simulink model "Srm_dtc"  (Simulink 8.5)
settings: Solver=FixedStepDiscrete  StartTime=0.0  StopTime=1  FixedStep=Ts  RelTol=1e-3  AbsTol=1e-5
PreLoadFcn:
  | Ts=1e-5;
  | load srm64_60kw
undefined symbols (not defined in the file or in its folder): find_system, magnitude
libraries: powerlib x15, simulink x1
Description:
  | Copyright 2008-2010 The MathWorks, Inc.
settings Model: Creator=MathWorks  LastModifiedBy=think0404  ExtModeAutoUpdateStatusClock=off
settings DataIOCC: SignalLoggingName=sigsOut
settings OptimizationCC: InitFltsAndDblsToZero=on
settings DebuggingCC: CheckExecutionContextPreStartOutputMsg=on  CheckExecutionContextRuntimeOutputMsg=on  SignalResolutionControl=TryResolveAllWithWarning  MultiTaskDSMMsg=warning  MultiTaskCondExecSysMsg=none  FcnCallInpInsideContextMsg=UseLocalSettings
settings HardwareCC: TargetUnknown=on

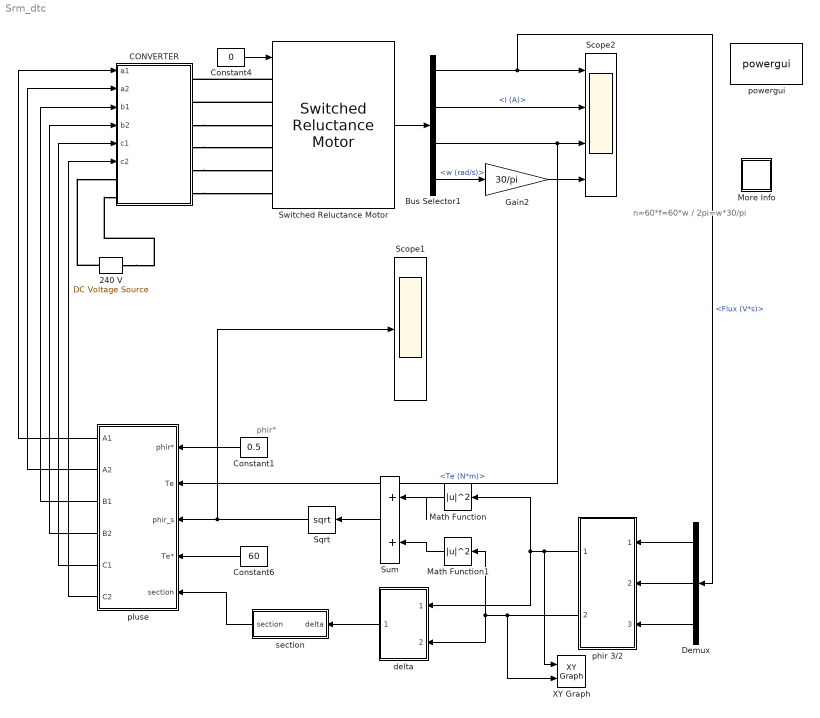
== system Srm_dtc ==
  note: phir*
  note: n=60*f=60*w / 2pi=w*30/pi
  " phir 3/2" : Subsystem
  240 V : powerlib/Electrical Sources/DC Voltage Source  Amplitude=300  Measurements=None
  Bus Selector1 : BusSelector  OutputSignals=Flux (V*s),I (A),Te (N*m),w (rad/s)
  CONVERTER : Subsystem  LoadFcn=find_system(gcs,'FollowLinks', 'on', 'LookUnderMasks', 'all');
  Constant1 : Constant  Value=0.5
  Constant4 : Constant  Value=0
  Constant6 : Constant  Value=60
  Demux : Demux  Outputs=3
  Gain2 : Gain  Gain=30/pi  SaturateOnIntegerOverflow=on  OutDataTypeStr=Inherit: Same as input  ParamDataTypeStr=Inherit: Same as input
  Math Function : Math  Operator=magnitude^2  SaturateOnIntegerOverflow=on
  Math Function1 : Math  Operator=magnitude^2  SaturateOnIntegerOverflow=on
  More Info : Subsystem  Description=asb
      settings: OpenFcn=showdemo(bdroot(gcb))
      mask Display: disp('?')
  Scope1 : Scope
      settings: TimeRange=0.1  YMin=-0.05  YMax=0.55  SaveName=VI1  Decimation=10
  Scope2 : Scope  NumInputPorts=4
      settings: TimeRange=0.1  YMin=-0.05~-100~-20~-10  YMax=0.55~800~70~90  SaveName=VI  Decimation=10
  Sqrt : Sqrt  SaturateOnIntegerOverflow=on
  Sum : Sum  Inputs=|++
  Switched Reluctance Motor : powerlib/Machines/Switched Reluctance Motor  MachineType=6/4  StatorResistance=0.05  Inertia=0.05  Friction=0.02  InitialSpeed=[0,0]  TsPowergui=0  TsBlock=-1  MachineModel=Generic model  Lq=0.67e-3  Ld=23.6e-3  Lsat=0.15e-3  MaximumCurrent=450  MaximumFluxLinkage=0.486  Source=MAT-file  MagnetisationCharacteristic='srm64_60kw.mat'  RotorAngleVector=[0 10 20 30 40 45]  StatorCurrentVector=0:25:450  PlotCurves=off
  XY Graph : simulink/Sinks/XY Graph  xmin=-1  xmax=1  ymin=-1  ymax=1  st=-1
  "delta " : Subsystem
  pluse : Subsystem
  powergui : powerlib/powergui  Priority=2  SimulationMode=Discrete  SolverType=Tustin/Backward Euler (TBE)  SampleTime=Ts  frequency=60  SPID=off  DisableSnubberDevices=off  DisableRonSwitches=off  DisableVfSwitches=off  SwTol=0  DisplayEquations=off  Interpol=off  methode=off  Ts=0  FunctionMessages=off  echomessages=off  HookPort=off  EnableUseOfTLC=off  x0status=blocks  frequencyindice=0  Pbase=100e6  ErrMax=1e-4  Iterations=50  UnitsV=kV  UnitsW=MW  buscounter=0  RestoreLinks=warning  ResistiveCurrentMeasurement=off  Frange=[0:2:500]  Ylog=off  Xlog=on  ShowGrid=off  save=off  variable=ZData  structure=0  ZoomFFT=on  StartTime=0.0  cycles=1  DisplayStyle=1  fundamental=60  FreqAxis=off  MaxFrequency=1000  frequencyindicesteady=1  RmsSteady=1  display=off
  "section " : Subsystem
  wires:
  Constant4/1 -> Switched Reluctance Motor/1
  Switched Reluctance Motor/1 -> Bus Selector1/1
  Bus Selector1/1 -> Scope2/1, Demux/1  "<Flux (V*s)>"
  Bus Selector1/2 -> Scope2/2  "<I (A)>"
  Bus Selector1/3 -> Scope2/3, pluse/2(Te)  "<Te (N*m)>"
  Gain2/1 -> Scope2/4
  Bus Selector1/4 -> Gain2/1  "<w (rad/s)>"
  Demux/1 -> " phir 3/2"/1(phir_a)
  Demux/2 -> " phir 3/2"/2(phir_b)
  Demux/3 -> " phir 3/2"/3(phir_c)
  " phir 3/2"/1(phir_alpha) -> Math Function/1, "delta "/1(phir_alpha), XY Graph/1
  " phir 3/2"/2(phir_beta) -> Math Function1/1, "delta "/2(phir_beta), XY Graph/2
  Math Function/1 -> Sum/1
  Math Function1/1 -> Sum/2
  Sum/1 -> Sqrt/1
  "delta "/1(delta) -> "section "/1(delta)
  Sqrt/1 -> pluse/3(phir_s), Scope1/1
  Constant1/1 -> pluse/1(phir*)
  Constant6/1 -> pluse/4(Te*)
  "section "/1(section) -> pluse/5(section)
  pluse/1(A1) -> CONVERTER/1(a1)
  pluse/2(A2) -> CONVERTER/2(a2)
  pluse/3(B1) -> CONVERTER/3(b1)
  pluse/4(B2) -> CONVERTER/4(b2)
  pluse/5(C1) -> CONVERTER/5(c1)
  pluse/6(C2) -> CONVERTER/6(c2)
  connections:
  Switched Reluctance Motor/LConn1 -- CONVERTER/RConn1
  Switched Reluctance Motor/LConn2 -- CONVERTER/RConn2
  CONVERTER/RConn3 -- Switched Reluctance Motor/LConn3
  CONVERTER/RConn4 -- Switched Reluctance Motor/LConn4
  CONVERTER/RConn5 -- Switched Reluctance Motor/LConn5
  CONVERTER/RConn6 -- Switched Reluctance Motor/LConn6
  240 V/RConn1 -- CONVERTER/LConn1
  240 V/LConn1 -- CONVERTER/LConn2

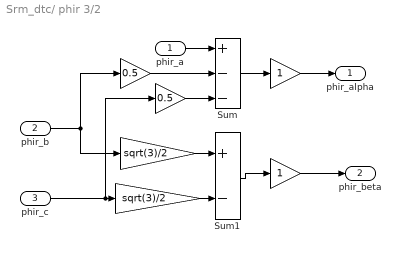
== system Srm_dtc/ phir 3/2 ==
  phir_a : Inport
  phir_b : Inport  Port=2
  phir_c : Inport  Port=3
  " " : Gain  Gain=0.5
  "   " : Gain  Gain=0.5
  "    " : Gain  Gain=sqrt(3)/2
  "     " : Gain  Gain=sqrt(3)/2
  "          " : Gain
  "              " : Gain
  Sum : Sum  Inputs=+--
  Sum1 : Sum  Inputs=+-
  phir_alpha : Outport
  phir_beta : Outport  Port=2
  wires:
  phir_a/1 -> Sum/1
  " "/1 -> Sum/2
  "   "/1 -> Sum/3
  "     "/1 -> Sum1/1
  "    "/1 -> Sum1/2
  phir_b/1 -> " "/1, "     "/1
  phir_c/1 -> "   "/1, "    "/1
  Sum/1 -> "          "/1
  Sum1/1 -> "              "/1
  "          "/1 -> phir_alpha/1
  "              "/1 -> phir_beta/1

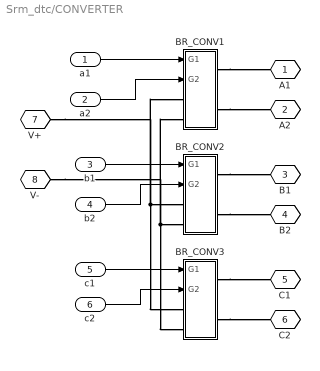
== system Srm_dtc/CONVERTER ==
  a1 : Inport
  a2 : Inport  Port=2
  b1 : Inport  Port=3
  b2 : Inport  Port=4
  c1 : Inport  Port=5
  c2 : Inport  Port=6
  BR_CONV1 : Subsystem
  BR_CONV2 : Subsystem
  BR_CONV3 : Subsystem
  A1 : PMIOPort  Tag=PMCPort  Port=1  Side=Right
  A2 : PMIOPort  Tag=PMCPort  Port=2  Side=Right
  B1 : PMIOPort  Tag=PMCPort  Port=3  Side=Right
  B2 : PMIOPort  Tag=PMCPort  Port=4  Side=Right
  C1 : PMIOPort  Tag=PMCPort  Port=5  Side=Right
  C2 : PMIOPort  Tag=PMCPort  Port=6  Side=Right
  V+ : PMIOPort  Tag=PMCPort  Port=7  Side=Left
  V- : PMIOPort  Tag=PMCPort  Port=8  Side=Left
  wires:
  a1/1 -> BR_CONV1/1(G1)
  a2/1 -> BR_CONV1/2(G2)
  b1/1 -> BR_CONV2/1(G1)
  b2/1 -> BR_CONV2/2(G2)
  c1/1 -> BR_CONV3/1(G1)
  c2/1 -> BR_CONV3/2(G2)
  connections:
  BR_CONV3/RConn2 -- C2/RConn1
  BR_CONV3/RConn1 -- C1/RConn1
  BR_CONV2/RConn2 -- B2/RConn1
  BR_CONV2/RConn1 -- B1/RConn1
  BR_CONV1/RConn2 -- A2/RConn1
  BR_CONV1/RConn1 -- A1/RConn1
  V+/RConn1 -- BR_CONV1/LConn1 -- BR_CONV2/LConn1 -- BR_CONV3/LConn1
  V-/RConn1 -- BR_CONV1/LConn2 -- BR_CONV2/LConn2 -- BR_CONV3/LConn2

== system Srm_dtc/More Info ==

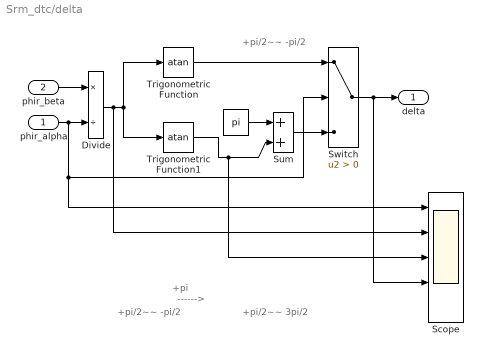
== system Srm_dtc/delta  ==
  note: +pi/2~~ -pi/2
  note: +pi/2~~ 3pi/2
  note: +pi/2~~ -pi/2
  note: ------>
  note: +pi
  phir_alpha : Inport
  phir_beta : Inport  Port=2
  " " : Constant  Value=pi
  Divide : Product  Inputs=*/
  Scope : Scope  NumInputPorts=5
      settings: YMin=-0.25~-1.75e+016~-2~-2~-1  YMax=1.25~2.5e+015~2~5~1  SaveName=ScopeData10
  Sum : Sum
  Switch : Switch  Criteria=u2 > Threshold
  Trigonometric Function : Trigonometry  Operator=atan
  Trigonometric Function1 : Trigonometry  Operator=atan
  delta : Outport
  wires:
  phir_alpha/1 -> Divide/2, Switch/2, Scope/1
  phir_beta/1 -> Divide/1
  Divide/1 -> Trigonometric Function/1, Trigonometric Function1/1, Scope/2
  " "/1 -> Sum/1
  Sum/1 -> Switch/3
  Switch/1 -> delta/1, Scope/4
  Trigonometric Function/1 -> Switch/1
  Trigonometric Function1/1 -> Sum/2, Scope/3

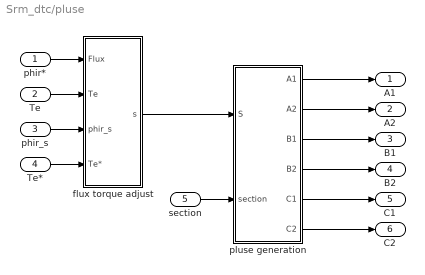
== system Srm_dtc/pluse ==
  phir* : Inport
  Te : Inport  Port=2
  phir_s : Inport  Port=3
  Te* : Inport  Port=4
  section : Inport  Port=5
  flux torque adjust : Subsystem
  pluse generation : Subsystem
  A1 : Outport
  A2 : Outport  Port=2
  B1 : Outport  Port=3
  B2 : Outport  Port=4
  C1 : Outport  Port=5
  C2 : Outport  Port=6
  wires:
  phir*/1 -> flux torque adjust/1(Flux)
  Te/1 -> flux torque adjust/2(Te)
  phir_s/1 -> flux torque adjust/3(phir_s)
  Te*/1 -> flux torque adjust/4(Te*)
  section/1 -> pluse generation/2(section)
  flux torque adjust/1(s) -> pluse generation/1(S)
  pluse generation/1(A1) -> A1/1
  pluse generation/2(A2) -> A2/1
  pluse generation/3(B1) -> B1/1
  pluse generation/4(B2) -> B2/1
  pluse generation/5(C1) -> C1/1
  pluse generation/6(C2) -> C2/1

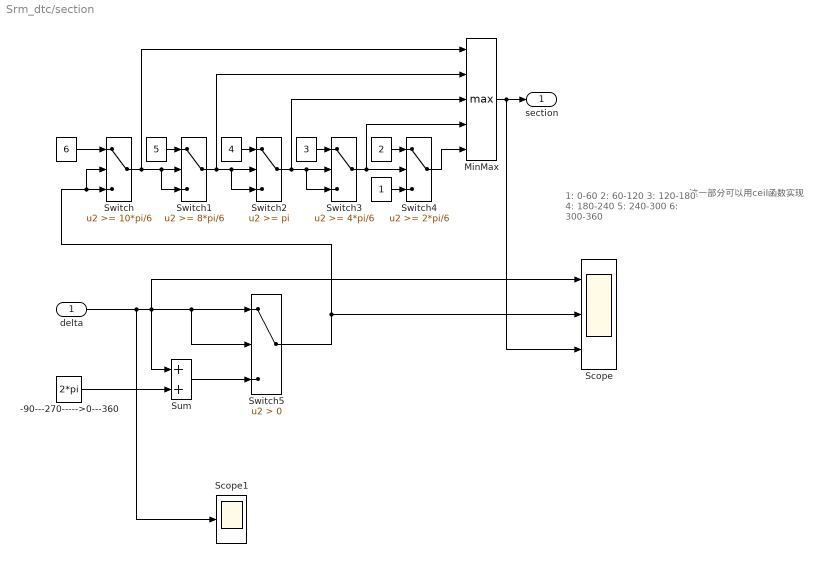
== system Srm_dtc/section  ==
  note: 这一部分可以用ceil函数实现
  note: 1:     0-60
      | 2:   60-120
      | 3:  120-180
      | 4:  180-240
      | 5:  240-300
      | 6:  300-360
  delta : Inport
  " " : Constant  Value=3
  "  " : Constant  Value=6
  "   " : Constant  Value=4
  "     " : Constant
  "      " : Constant  Value=5
  "       " : Constant  Value=2
  " -90---270----->0---360" : Constant  Value=2*pi
  MinMax : MinMax  Function=max  Inputs=5
  Scope : Scope  NumInputPorts=3
      settings: YMin=-5~-5~-5  YMax=5~5~5  SaveName=ScopeData2
  Scope1 : Scope
      settings: TimeRange=0.1  YMin=-2  SaveName=VI2  Decimation=10
  Sum : Sum
  Switch : Switch  Threshold=10*pi/6
  Switch1 : Switch  Threshold=8*pi/6
  Switch2 : Switch  Threshold=pi
  Switch3 : Switch  Threshold=4*pi/6
  Switch4 : Switch  Threshold=2*pi/6
  Switch5 : Switch  Criteria=u2 > Threshold
  section : Outport
  wires:
  "  "/1 -> Switch/1
  Switch/1 -> MinMax/1, Switch1/2, Switch1/3
  "      "/1 -> Switch1/1
  Switch1/1 -> MinMax/2, Switch2/2, Switch2/3
  "   "/1 -> Switch2/1
  Switch2/1 -> MinMax/3, Switch3/2, Switch3/3
  " "/1 -> Switch3/1
  Switch3/1 -> Switch4/2, MinMax/4
  "       "/1 -> Switch4/1
  Switch4/1 -> MinMax/5
  "     "/1 -> Switch4/3
  MinMax/1 -> section/1, Scope/3
  delta/1 -> Scope1/1, Switch5/1, Switch5/2, Sum/1, Scope/1
  " -90---270----->0---360"/1 -> Sum/2
  Sum/1 -> Switch5/3
  Switch5/1 -> Switch/3, Switch/2, Scope/2

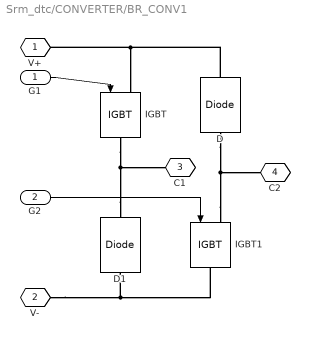
== system Srm_dtc/CONVERTER/BR_CONV1 ==
  G1 : Inport
  G2 : Inport  Port=2
  D : powerlib/Power Electronics/Diode  Ron=1e-3  Lon=0  Vf=0.8  IC=0  UseSnubber=off  Rs=1000  Cs=inf  Measurements=off
  D1 : powerlib/Power Electronics/Diode  Ron=1e-3  Lon=0  Vf=0.8  IC=0  UseSnubber=off  Rs=1000  Cs=inf  Measurements=off
  IGBT : powerlib/Power Electronics/IGBT  Ron=1e-3  Lon=0  Vf=1  Tf=0  Tt=0  IC=0  Rs=200  Cs=0.1e-6  Measurements=off
  IGBT1 : powerlib/Power Electronics/IGBT  Ron=1e-3  Lon=0  Vf=1  Tf=0  Tt=0  IC=0  Rs=200  Cs=0.1e-6  Measurements=off
  V+ : PMIOPort  Tag=PMCPort  Port=1  Side=Left
  V- : PMIOPort  Tag=PMCPort  Port=2  Side=Left
  C1 : PMIOPort  Tag=PMCPort  Port=3  Side=Right
  C2 : PMIOPort  Tag=PMCPort  Port=4  Side=Right
  wires:
  G2/1 -> IGBT1/1
  G1/1 -> IGBT/1
  connections:
  D1/LConn1 -- V-/RConn1 -- IGBT1/RConn1
  IGBT1/LConn1 -- D/LConn1 -- C2/RConn1
  D1/RConn1 -- IGBT/RConn1 -- C1/RConn1
  D/RConn1 -- V+/RConn1 -- IGBT/LConn1

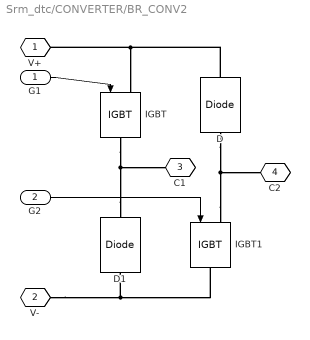
== system Srm_dtc/CONVERTER/BR_CONV2 ==
  G1 : Inport
  G2 : Inport  Port=2
  D : powerlib/Power Electronics/Diode  Ron=1e-3  Lon=0  Vf=0.8  IC=0  UseSnubber=off  Rs=1000  Cs=inf  Measurements=off
  D1 : powerlib/Power Electronics/Diode  Ron=1e-3  Lon=0  Vf=0.8  IC=0  UseSnubber=off  Rs=1000  Cs=inf  Measurements=off
  IGBT : powerlib/Power Electronics/IGBT  Ron=1e-3  Lon=0  Vf=1  Tf=0  Tt=0  IC=0  Rs=200  Cs=0.1e-6  Measurements=off
  IGBT1 : powerlib/Power Electronics/IGBT  Ron=1e-3  Lon=0  Vf=1  Tf=0  Tt=0  IC=0  Rs=200  Cs=0.1e-6  Measurements=off
  V+ : PMIOPort  Tag=PMCPort  Port=1  Side=Left
  V- : PMIOPort  Tag=PMCPort  Port=2  Side=Left
  C1 : PMIOPort  Tag=PMCPort  Port=3  Side=Right
  C2 : PMIOPort  Tag=PMCPort  Port=4  Side=Right
  wires:
  G2/1 -> IGBT1/1
  G1/1 -> IGBT/1
  connections:
  D1/LConn1 -- V-/RConn1 -- IGBT1/RConn1
  IGBT1/LConn1 -- D/LConn1 -- C2/RConn1
  D1/RConn1 -- IGBT/RConn1 -- C1/RConn1
  D/RConn1 -- V+/RConn1 -- IGBT/LConn1

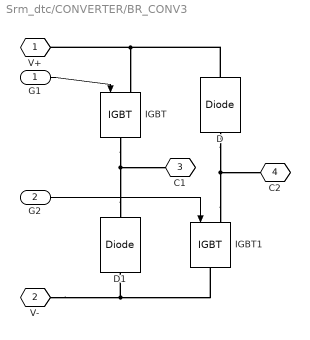
== system Srm_dtc/CONVERTER/BR_CONV3 ==
  G1 : Inport
  G2 : Inport  Port=2
  D : powerlib/Power Electronics/Diode  Ron=1e-3  Lon=0  Vf=0.8  IC=0  UseSnubber=off  Rs=1000  Cs=inf  Measurements=off
  D1 : powerlib/Power Electronics/Diode  Ron=1e-3  Lon=0  Vf=0.8  IC=0  UseSnubber=off  Rs=1000  Cs=inf  Measurements=off
  IGBT : powerlib/Power Electronics/IGBT  Ron=1e-3  Lon=0  Vf=1  Tf=0  Tt=0  IC=0  Rs=200  Cs=0.1e-6  Measurements=off
  IGBT1 : powerlib/Power Electronics/IGBT  Ron=1e-3  Lon=0  Vf=1  Tf=0  Tt=0  IC=0  Rs=200  Cs=0.1e-6  Measurements=off
  V+ : PMIOPort  Tag=PMCPort  Port=1  Side=Left
  V- : PMIOPort  Tag=PMCPort  Port=2  Side=Left
  C1 : PMIOPort  Tag=PMCPort  Port=3  Side=Right
  C2 : PMIOPort  Tag=PMCPort  Port=4  Side=Right
  wires:
  G2/1 -> IGBT1/1
  G1/1 -> IGBT/1
  connections:
  D1/LConn1 -- V-/RConn1 -- IGBT1/RConn1
  IGBT1/LConn1 -- D/LConn1 -- C2/RConn1
  D1/RConn1 -- IGBT/RConn1 -- C1/RConn1
  D/RConn1 -- V+/RConn1 -- IGBT/LConn1

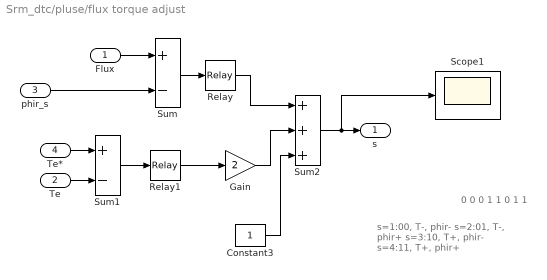
== system Srm_dtc/pluse/flux torque adjust ==
  note: 0 0
      | 0 1
      | 1 0
      | 1 1
  note: s=1:00, T-,  phir-
      | s=2:01, T-,  phir+
      | s=3:10, T+,  phir-
      | s=4:11, T+,  phir+
  Flux : Inport
  Te : Inport  Port=2
  phir_s : Inport  Port=3
  Te* : Inport  Port=4
  Constant3 : Constant
  Gain : Gain  Gain=2
  Relay : Relay  OnSwitchValue=0.005  OffSwitchValue=-0.005
  Relay1 : Relay  OnSwitchValue=0.01  OffSwitchValue=-0.01
  Scope1 : Scope
      settings: TimeRange=0.1  YMin=-0.05  YMax=0.55  SaveName=VI3  Decimation=10
  Sum : Sum  Inputs=+-
  Sum1 : Sum  Inputs=+-
  Sum2 : Sum  Inputs=+++
  s : Outport
  wires:
  Flux/1 -> Sum/1
  phir_s/1 -> Sum/2
  Sum/1 -> Relay/1
  Te*/1 -> Sum1/1
  Te/1 -> Sum1/2
  Sum1/1 -> Relay1/1
  Relay1/1 -> Gain/1
  Relay/1 -> Sum2/1
  Gain/1 -> Sum2/2
  Sum2/1 -> Scope1/1, s/1
  Constant3/1 -> Sum2/3

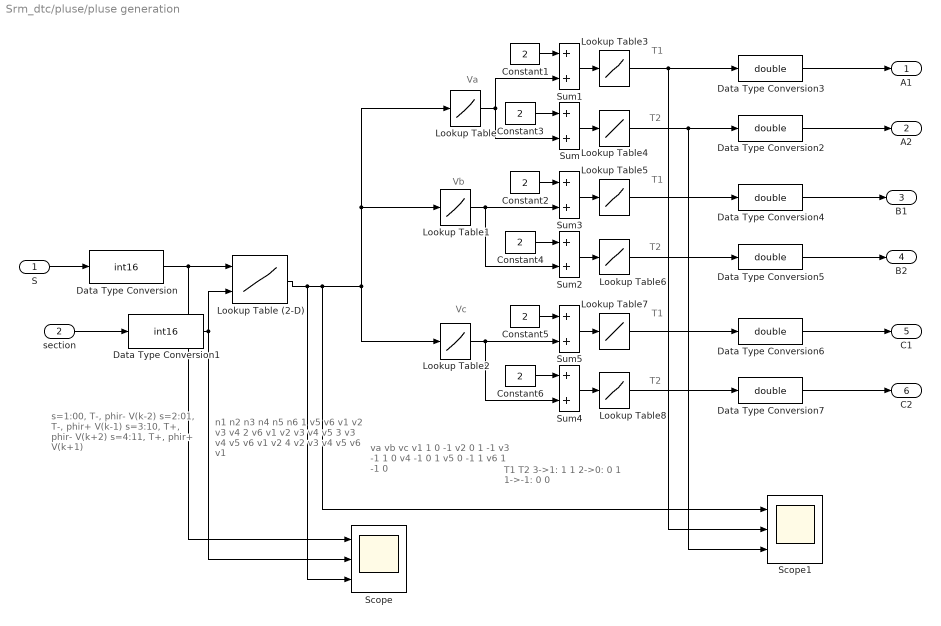
== system Srm_dtc/pluse/pluse generation ==
  note: n1   n2  n3  n4   n5  n6
      |    1  v5   v6   v1   v2   v3   v4
      |    2  v6   v1   v2   v3   v4   v5
      |    3  v3   v4   v5   v6   v1   v2
      |   4  v2   v3   v4   v5   v6   v1
  note: s=1:00, T-,  phir-     V(k-2)
      | s=2:01, T-,  phir+     V(k-1)
      | s=3:10, T+,  phir-     V(k+2)
      | s=4:11, T+,  phir+     V(k+1)
  note: va    vb     vc
      | v1  1     0     -1
      | v2  0     1     -1
      | v3  -1     1     0
      | v4  -1     0     1
      | v5  0     -1    1
      | v6  1     -1     0
  note: T1    T2
      | 3->1:  1      1
      | 2->0:  0      1
      | 1->-1:  0      0
  note: Va
  note: Vb
  note: Vc
  note: T1
  note: T2
  note: T1
  note: T2
  note: T1
  note: T2
  S : Inport
  section : Inport  Port=2
  Constant{1..6} (6 alike) : Constant  Value=2
  Data Type Conversion : DataTypeConversion  OutDataTypeStr=int16
  Data Type Conversion1 : DataTypeConversion  OutDataTypeStr=int16
  Data Type Conversion{2..7} (6 alike) : DataTypeConversion  OutDataTypeStr=double
  Lookup Table (2-D) : Lookup2D  RowIndex=[1:4]  ColumnIndex=[1:6]  Table=[5 6 1 2 3 4;6 1 2 3 4 5;3 4 5 6 1 2;2 3 4 5 6 1]
  Lookup Table : Lookup  InputValues=[1:6]  Table=[1 0 -1 -1 0 1]
  Lookup Table1 : Lookup  InputValues=[1:6]  Table=[0 1 1 0 -1 -1]
  Lookup Table2 : Lookup  InputValues=[1:6]  Table=[-1 -1 0 1 1 0]
  Lookup Table3 : Lookup  InputValues=[1:3]  Table=[0 0 1]
  Lookup Table4 : Lookup  InputValues=[1:3]  Table=[0 1 1]
  Lookup Table5 : Lookup  InputValues=[1:3]  Table=[0 0 1]
  Lookup Table6 : Lookup  InputValues=[1:3]  Table=[0 1 1]
  Lookup Table7 : Lookup  InputValues=[1:3]  Table=[0 0 1]
  Lookup Table8 : Lookup  InputValues=[1:3]  Table=[0 1 1]
  Scope : Scope  NumInputPorts=3
      settings: YMin=4~1~1  YMax=4~6~6
  Scope1 : Scope  NumInputPorts=3
      settings: YMin=1~0~0  YMax=6~1~1
  Sum{,1..5} (6 alike) : Sum
  A1 : Outport
  A2 : Outport  Port=2
  B1 : Outport  Port=3
  B2 : Outport  Port=4
  C1 : Outport  Port=5
  C2 : Outport  Port=6
  wires:
  S/1 -> Data Type Conversion/1
  section/1 -> Data Type Conversion1/1
  Data Type Conversion/1 -> Lookup Table (2-D)/1, Scope/1
  Data Type Conversion1/1 -> Lookup Table (2-D)/2, Scope/2
  Lookup Table (2-D)/1 -> Scope/3, Lookup Table2/1, Lookup Table/1, Lookup Table1/1, Scope1/1
  Constant1/1 -> Sum1/1
  Sum1/1 -> Lookup Table3/1
  Constant3/1 -> Sum/1
  Sum/1 -> Lookup Table4/1
  Lookup Table/1 -> Sum1/2, Sum/2
  Constant2/1 -> Sum3/1
  Sum3/1 -> Lookup Table5/1
  Constant4/1 -> Sum2/1
  Sum2/1 -> Lookup Table6/1
  Lookup Table1/1 -> Sum2/2, Sum3/2
  Constant5/1 -> Sum5/1
  Sum5/1 -> Lookup Table7/1
  Constant6/1 -> Sum4/1
  Sum4/1 -> Lookup Table8/1
  Lookup Table2/1 -> Sum5/2, Sum4/2
  Lookup Table3/1 -> Data Type Conversion3/1, Scope1/2
  Lookup Table4/1 -> Data Type Conversion2/1, Scope1/3
  Lookup Table5/1 -> Data Type Conversion4/1
  Lookup Table6/1 -> Data Type Conversion5/1
  Lookup Table7/1 -> Data Type Conversion6/1
  Lookup Table8/1 -> Data Type Conversion7/1
  Data Type Conversion3/1 -> A1/1
  Data Type Conversion2/1 -> A2/1
  Data Type Conversion4/1 -> B1/1
  Data Type Conversion5/1 -> B2/1
  Data Type Conversion6/1 -> C1/1
  Data Type Conversion7/1 -> C2/1
